simulink model "Flyback Simulink Model"  (R2019b)
settings: Solver=VariableStepAuto  StartTime=0.0  StopTime=5  FixedStep=0.0001  RelTol=1e-3
undefined symbols (not defined in the file): plecs
libraries: simulink x6, plecslib_extras2 x3, simulink_extras x2
settings Model: Creator=jeffl  LastModifiedBy=jeffl
settings SolverCC: ZeroCrossAlgorithm=Adaptive
settings DebuggingCC: IgnoredZcDiagnostic=none

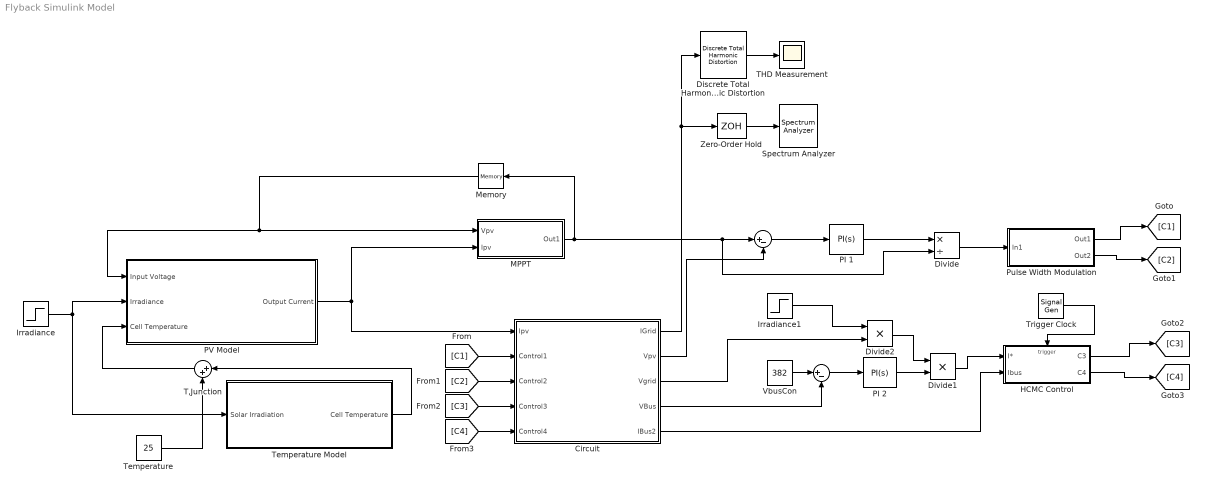
== system Flyback Simulink Model ==
  " " : Sum  Inputs=|+-
  "   " : Sum  Inputs=|+-
  Circuit : Subsystem  LoadFcn=plecs('sl', 200);  InitFcn=plecs('sl', 214);  StartFcn=plecs('sl', 208);  StopFcn=plecs('sl', 209);  mask(PlecsCircuit){PLECSData=<binary blob, 6696 chars, not shown>}
      mask prompts: PLECSData "PLECS Data (Do not delete or modify!)"
      mask init:
      | % PLACE CUSTOM INITIALIZATIONS ABOVE
      | % DO NOT REMOVE
      | plecs('sl', 215);
      | % DO NOT REMOVE
      settings: CopyFcn=plecs('sl', 203);  DeleteFcn=plecs('sl', 205);  UndoDeleteFcn=plecs('sl', 206);  PreSaveFcn=plecs('sl', 211);  PostSaveFcn=plecs('sl', 201);  NameChangeFcn=plecs('sl', 210);  DestroyFcn=plecs('sl', 207);  PreCopyFcn=plecs('sl', 216);  OpenFcn=plecs('sl', 202);  ErrorFcn=plerrorfcn
      mask Help: web(['file:///' fullfile(plecsdoc, 'creatingacircuit.html')])
      mask Display: disp('PLECS\nCircuit')
  Discrete Total Harmonic Distortion : plecslib_extras2/Discrete Analysis/Discrete Total Harmonic Distortion  Ts=1/600  samples=10
      settings: SourceProductName=PLECS Extras
  Divide : Product  Inputs=*/
  Divide1 : Product  Inputs=**
  Divide2 : Product  Inputs=**
  HCMC Control : Subsystem
  Irradiance : Step  Before=1000  After=1000  SampleTime=0
  Irradiance1 : Step  Before=1/220  After=1/245  SampleTime=0
  MPPT : Subsystem
  Memory : Memory  InitialCondition=28
  PI 1 : simulink/Continuous/PID Controller  Controller=PI  Form=Parallel  TimeDomain=Continuous-time  SampleTime=-1  IntegratorMethod=Forward Euler  FilterMethod=Forward Euler  ControllerParametersSource=internal  P=-2  I=-2  D=0  UseFilter=on  N=100  TunerSelectOption=Transfer Function Based (PID Tuner App)  InitialConditionSource=internal  InitialConditionForIntegrator=0  InitialConditionForFilter=0  DifferentiatorICPrevScaledInput=0  ExternalReset=none  TrackingMode=off  Kt=1  LimitOutput=off  UpperSaturationLimit=inf  LowerSaturationLimit=-inf  LinearizeAsGain=on  AntiWindupMode=none  Kb=1  POutMin=[]  POutMax=[]  IOutMin=[]  IOutMax=[]  DOutMin=[]  DOutMax=[]  NOutMin=[]  NOutMax=[]  SumOutMin=[]  SumOutMax=[]  SaturationOutMin=[]  SaturationOutMax=[]  PParamMin=[]  PParamMax=[]  IParamMin=[]  IParamMax=[]  DParamMin=[]  DParamMax=[]  NParamMin=[]  NParamMax=[]  KbParamMin=[]  KbParamMax=[]  KtParamMin=[]  KtParamMax=[]  KbOutMin=[]  KbOutMax=[]  KtOutMin=[]  KtOutMax=[]  IntegratorOutMin=[]  IntegratorOutMax=[]  FilterOutMin=[]  FilterOutMax=[]  SumI1OutMin=[]  SumI1OutMax=[]  SumI2OutMin=[]  SumI2OutMax=[]  SumI3OutMin=[]  SumI3OutMax=[]  SumI4OutMin=[]  SumI4OutMax=[]  SumDOutMin=[]  SumDOutMax=[]  DifferentiatorOutMin=[]  DifferentiatorOutMax=[]  FilterDiffOutCoefMin=[]  FilterDiffOutCoefMax=[]  ReciprocalOutMin=[]  ReciprocalOutMax=[]  SumDenOutMin=[]  SumDenOutMax=[]  SumNumOutMin=[]  SumNumOutMax=[]  DivideOutMin=[]  DivideOutMax=[]  IntegratorContinuousStateAttributes=''  IntegratorStateMustResolveToSignalObject=off  IntegratorRTWStateStorageClass=Auto  FilterContinuousStateAttributes=''  FilterStateMustResolveToSignalObject=off  FilterRTWStateStorageClass=Auto  ParallelPVariant=InternalParameters  IdealPVariant=Disabled  IVariant=InternalParameters  DVariant=Disabled  IntegratorVariant=Continuous  SatVariant=Disabled  AWVariant=Passthrough  PCopyVariant=Disabled  TRVariant=Disabled  FdbkBlocksVariant=Forward  IdealPFdbkVariant=Disabled  SatFdbkVariant=Disabled  DerivativeFilterVariant=Disabled  NVariant=Disabled  NCopyVariant=Disabled_SignalSpec  FilterICVariant=Disabled  IntegratorICVariant=InternalICs  ExternalResetVariant=Disabled  TRSumVariant=Passthrough  SumFdbkVariant=Disabled  SumVariant=Sum_PI
  PI 2 : simulink/Continuous/PID Controller  Controller=PI  Form=Parallel  TimeDomain=Continuous-time  SampleTime=-1  IntegratorMethod=Forward Euler  FilterMethod=Forward Euler  ControllerParametersSource=internal  P=1/10  I=0.5  D=0  UseFilter=on  N=100  TunerSelectOption=Transfer Function Based (PID Tuner App)  InitialConditionSource=internal  InitialConditionForIntegrator=0  InitialConditionForFilter=0  DifferentiatorICPrevScaledInput=0  ExternalReset=none  TrackingMode=off  Kt=1  LimitOutput=off  UpperSaturationLimit=inf  LowerSaturationLimit=-inf  LinearizeAsGain=on  AntiWindupMode=none  Kb=1  POutMin=[]  POutMax=[]  IOutMin=[]  IOutMax=[]  DOutMin=[]  DOutMax=[]  NOutMin=[]  NOutMax=[]  SumOutMin=[]  SumOutMax=[]  SaturationOutMin=[]  SaturationOutMax=[]  PParamMin=[]  PParamMax=[]  IParamMin=[]  IParamMax=[]  DParamMin=[]  DParamMax=[]  NParamMin=[]  NParamMax=[]  KbParamMin=[]  KbParamMax=[]  KtParamMin=[]  KtParamMax=[]  KbOutMin=[]  KbOutMax=[]  KtOutMin=[]  KtOutMax=[]  IntegratorOutMin=[]  IntegratorOutMax=[]  FilterOutMin=[]  FilterOutMax=[]  SumI1OutMin=[]  SumI1OutMax=[]  SumI2OutMin=[]  SumI2OutMax=[]  SumI3OutMin=[]  SumI3OutMax=[]  SumI4OutMin=[]  SumI4OutMax=[]  SumDOutMin=[]  SumDOutMax=[]  DifferentiatorOutMin=[]  DifferentiatorOutMax=[]  FilterDiffOutCoefMin=[]  FilterDiffOutCoefMax=[]  ReciprocalOutMin=[]  ReciprocalOutMax=[]  SumDenOutMin=[]  SumDenOutMax=[]  SumNumOutMin=[]  SumNumOutMax=[]  DivideOutMin=[]  DivideOutMax=[]  IntegratorContinuousStateAttributes=''  IntegratorStateMustResolveToSignalObject=off  IntegratorRTWStateStorageClass=Auto  FilterContinuousStateAttributes=''  FilterStateMustResolveToSignalObject=off  FilterRTWStateStorageClass=Auto  ParallelPVariant=InternalParameters  IdealPVariant=Disabled  IVariant=InternalParameters  DVariant=Disabled  IntegratorVariant=Continuous  SatVariant=Disabled  AWVariant=Passthrough  PCopyVariant=Disabled  TRVariant=Disabled  FdbkBlocksVariant=Forward  IdealPFdbkVariant=Disabled  SatFdbkVariant=Disabled  DerivativeFilterVariant=Disabled  NVariant=Disabled  NCopyVariant=Disabled_SignalSpec  FilterICVariant=Disabled  IntegratorICVariant=InternalICs  ExternalResetVariant=Disabled  TRSumVariant=Passthrough  SumFdbkVariant=Disabled  SumVariant=Sum_PI
  PV Model : Subsystem
  Pulse Width Modulation : Subsystem
  "Spectrum Analyzer " : SpectrumAnalyzer
  T,Junction : Sum  Inputs=|++
  THD Measurement : Scope
  Temperature : Constant  Value=25
  Temperature Model : Subsystem
  Trigger Clock : SignalGenerator  WaveForm=square  Frequency=400e3  Units=rad/sec
  VbusCon : Constant  Value=382
  Zero-Order Hold : ZeroOrderHold  SampleTime=1/1500
  wires:
  MPPT/1(Out1) -> Memory/1, Divide/2, " "/1
  Memory/1 -> PV Model/1(Input Voltage), MPPT/1(Vpv)
  PV Model/1(Output Current) -> MPPT/2(Ipv), Circuit/1(Ipv)
  T,Junction/1 -> PV Model/3(Cell Temperature)
  Temperature/1 -> T,Junction/2
  Temperature Model/1(Cell Temperature) -> T,Junction/1
  Irradiance/1 -> PV Model/2(Irradiance), Temperature Model/1(Solar Irradiation)
  " "/1 -> PI 1/1
  PI 1/1 -> Divide/1
  Divide/1 -> Pulse Width Modulation/1(In1)
  Circuit/2(Vpv) -> " "/2
  Circuit/4(VBus) -> "   "/2
  VbusCon/1 -> "   "/1
  "   "/1 -> PI 2/1
  PI 2/1 -> Divide1/2
  Divide1/1 -> HCMC Control/1(I*)
  Circuit/5(IBus2) -> HCMC Control/2(Ibus)
  Trigger Clock/1 -> HCMC Control/Trigger
  Circuit/1(IGrid) -> Discrete Total Harmonic Distortion/1, Zero-Order Hold/1
  Discrete Total Harmonic Distortion/1 -> THD Measurement/1
  Zero-Order Hold/1 -> "Spectrum Analyzer "/1
  Pulse Width Modulation/1(Out1) -> [C1]
  Pulse Width Modulation/2(Out2) -> [C2]
  [C1] -> Circuit/2(Control1)
  [C2] -> Circuit/3(Control2)
  HCMC Control/2(C4) -> [C4]
  HCMC Control/1(C3) -> [C3]
  [C4] -> Circuit/5(Control4)
  [C3] -> Circuit/4(Control3)
  Circuit/3(Vgrid) -> Divide2/2
  Irradiance1/1 -> Divide2/1
  Divide2/1 -> Divide1/1

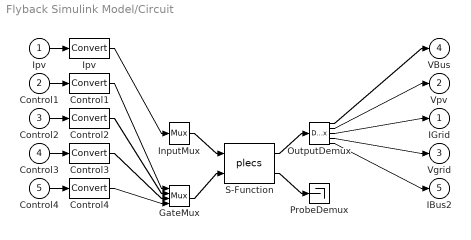
== system Flyback Simulink Model/Circuit ==
  Ipv : Inport  PortDimensions=1
  Control1 : Inport  Port=2  PortDimensions=1
  Control2 : Inport  Port=3  PortDimensions=1
  Control3 : Inport  Port=4  PortDimensions=1
  Control4 : Inport  Port=5  PortDimensions=1
  " Control1 " : DataTypeConversion  SaturateOnIntegerOverflow=on  RndMeth=Zero
  " Control2 " : DataTypeConversion  SaturateOnIntegerOverflow=on  RndMeth=Zero
  " Control3 " : DataTypeConversion  SaturateOnIntegerOverflow=on  RndMeth=Zero
  " Control4 " : DataTypeConversion  SaturateOnIntegerOverflow=on  RndMeth=Zero
  " GateMux " : Mux  Inputs=[ 1 1 1 1 ]
  " InputMux " : Mux  Inputs=[ 1 ]
  " Ipv " : DataTypeConversion  SaturateOnIntegerOverflow=on  RndMeth=Zero
  " OutputDemux " : Demux  Outputs=[ 1 1 1 1 1 ]
  " ProbeDemux " : Terminator
  " S-Function " : S-Function  FunctionName=plecs  SFunctionDeploymentMode=off  EnableBusSupport=off
  IGrid : Outport  PortDimensions=1
  Vpv : Outport  Port=2  PortDimensions=1
  Vgrid : Outport  Port=3  PortDimensions=1
  VBus : Outport  Port=4  PortDimensions=1
  IBus2 : Outport  Port=5  PortDimensions=1
  wires:
  " InputMux "/1 -> " S-Function "/1
  " GateMux "/1 -> " S-Function "/2
  " S-Function "/1 -> " OutputDemux "/1
  " S-Function "/2 -> " ProbeDemux "/1
  Ipv/1 -> " Ipv "/1
  " Ipv "/1 -> " InputMux "/1
  Control1/1 -> " Control1 "/1
  " Control1 "/1 -> " GateMux "/1
  Control2/1 -> " Control2 "/1
  " Control2 "/1 -> " GateMux "/2
  Control3/1 -> " Control3 "/1
  " Control3 "/1 -> " GateMux "/3
  Control4/1 -> " Control4 "/1
  " Control4 "/1 -> " GateMux "/4
  " OutputDemux "/1 -> VBus/1
  " OutputDemux "/2 -> Vpv/1
  " OutputDemux "/3 -> IGrid/1
  " OutputDemux "/4 -> Vgrid/1
  " OutputDemux "/5 -> IBus2/1

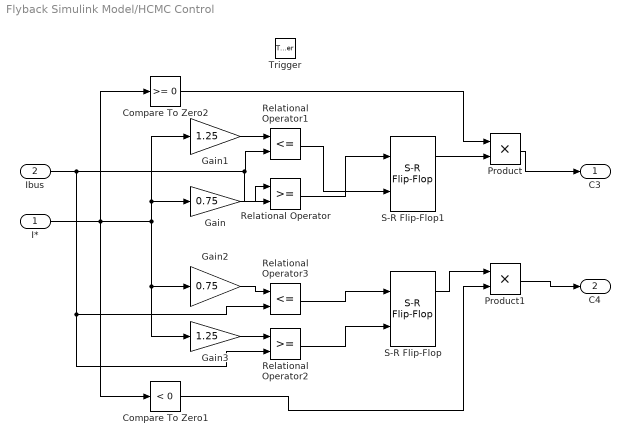
== system Flyback Simulink Model/HCMC Control ==
  I* : Inport
  Ibus : Inport  Port=2
  Trigger : TriggerPort  VariantControl=Variant  PortDimensions=1
  Compare To Zero1 : simulink/Logic and Bit Operations/Compare To Zero  relop=<  OutDataTypeStr=boolean  ZeroCross=off
  Compare To Zero2 : simulink/Logic and Bit Operations/Compare To Zero  relop=>=  OutDataTypeStr=boolean  ZeroCross=off
  Gain : Gain  Gain=0.75
  Gain1 : Gain  Gain=1.25
  Gain2 : Gain  Gain=0.75
  Gain3 : Gain  Gain=1.25
  Product : Product
  Product1 : Product
  Relational Operator : RelationalOperator  OutDataTypeStr=boolean  ZeroCross=off  RndMeth=Simplest
  Relational Operator1 : RelationalOperator  Operator=<=  OutDataTypeStr=boolean  ZeroCross=off  RndMeth=Simplest
  Relational Operator2 : RelationalOperator  OutDataTypeStr=boolean  ZeroCross=off  RndMeth=Simplest
  Relational Operator3 : RelationalOperator  Operator=<=  OutDataTypeStr=boolean  ZeroCross=off  RndMeth=Simplest
  S-R Flip-Flop : simulink_extras/Flip Flops/S-R Flip-Flop  initial_condition=0
  S-R Flip-Flop1 : simulink_extras/Flip Flops/S-R Flip-Flop  initial_condition=0
  C3 : Outport
  C4 : Outport  Port=2
  wires:
  I*/1 -> Gain3/1, Gain2/1, Gain1/1, Gain/1, Compare To Zero1/1, Compare To Zero2/1
  Gain1/1 -> Relational Operator1/1
  Compare To Zero2/1 -> Product/1
  Compare To Zero1/1 -> Product1/2
  S-R Flip-Flop/1 -> Product1/1
  S-R Flip-Flop1/1 -> Product/2
  Product/1 -> C3/1
  Product1/1 -> C4/1
  Ibus/1 -> Relational Operator/2, Relational Operator1/2, Relational Operator3/2, Relational Operator2/2
  Gain/1 -> Relational Operator/1
  Gain3/1 -> Relational Operator2/1
  Gain2/1 -> Relational Operator3/1
  Relational Operator/1 -> S-R Flip-Flop1/1
  Relational Operator1/1 -> S-R Flip-Flop1/2
  Relational Operator3/1 -> S-R Flip-Flop/1
  Relational Operator2/1 -> S-R Flip-Flop/2

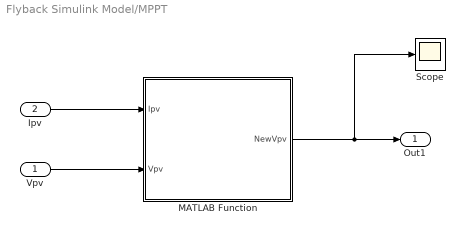
== system Flyback Simulink Model/MPPT ==
  Vpv : Inport
  Ipv : Inport  Port=2
  MATLAB Function : MATLAB Function  TreatAsAtomicUnit=on
  Scope : Scope
  Out1 : Outport  VectorParamsAs1DForOutWhenUnconnected=off
  wires:
  Ipv/1 -> MATLAB Function/1(Ipv)
  Vpv/1 -> MATLAB Function/2(Vpv)
  MATLAB Function/1(NewVpv) -> Scope/1, Out1/1

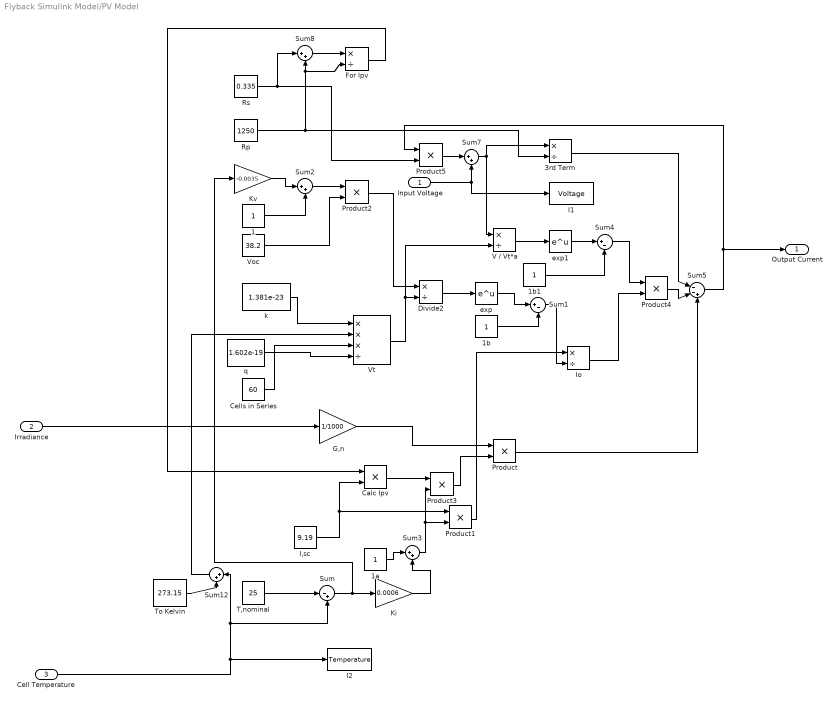
== system Flyback Simulink Model/PV Model ==
  Input Voltage : Inport
  Irradiance : Inport  Port=2
  Cell Temperature : Inport  Port=3
  1 : Constant
  1a : Constant
  1b : Constant
  1b1 : Constant
  3rd Term : Product  Inputs=*/
  Calc Ipv : Product
  Cells in Series : Constant  Value=60
  Divide2 : Product  Inputs=*/
  For Ipv : Product  Inputs=*/
  G,n : Gain  Gain=1/1000
  I,sc : Constant  Value=9.19
  I1 : ToWorkspace  VariableName=Voltage  SampleTime=-1
  I2 : ToWorkspace  VariableName=Temperature  SampleTime=-1
  Io : Product  Inputs=*/
  Ki : Gain  Gain=0.0006
  Kv : Gain  Gain=-0.0035
  Product{,1..5} (6 alike) : Product
  Rp : Constant  Value=1250
  Rs : Constant  Value=0.335
  Sum : Sum  Inputs=|-+
  Sum1 : Sum  Inputs=|+-
  Sum{2..3,7..8,12} (5 alike) : Sum  Inputs=|++
  Sum4 : Sum  Inputs=|+-
  Sum5 : Sum  Inputs=|--+
  T,nominal : Constant  Value=25
  To Kelvin : Constant  Value=273.15
  V / Vt*a : Product  Inputs=*/
  Voc : Constant  Value=38.2
  Vt : Product  Inputs=***/
  exp : Math  SaturateOnIntegerOverflow=on
  exp1 : Math  SaturateOnIntegerOverflow=on
  k : Constant  Value=1.381e-23
  q : Constant  Value=1.602e-19
  Output Current : Outport  VectorParamsAs1DForOutWhenUnconnected=off
  wires:
  1b1/1 -> Sum4/2
  I,sc/1 -> Product1/1, Calc Ipv/2
  Io/1 -> Product4/2
  Ki/1 -> Sum3/2
  exp/1 -> Sum1/1
  For Ipv/1 -> Calc Ipv/1
  3rd Term/1 -> Sum5/1
  Input Voltage/1 -> Sum7/2, I1/1
  To Kelvin/1 -> Sum12/2
  Sum7/1 -> V / Vt*a/1, 3rd Term/1
  Product2/1 -> Divide2/1
  Product/1 -> Sum5/3
  1/1 -> Sum2/2
  Rp/1 -> For Ipv/2, Sum8/2, 3rd Term/2
  Calc Ipv/1 -> Product3/1
  Product4/1 -> Sum5/2
  Sum1/1 -> Io/2
  Sum8/1 -> For Ipv/1
  1b/1 -> Sum1/2
  Sum12/1 -> Vt/2
  Divide2/1 -> exp/1
  V / Vt*a/1 -> exp1/1
  Voc/1 -> Product2/2
  Sum2/1 -> Product2/1
  Kv/1 -> Sum2/1
  1a/1 -> Sum3/1
  Cell Temperature/1 -> I2/1, Sum/2, Sum12/1
  Product3/1 -> Product/2
  G,n/1 -> Product/1
  k/1 -> Vt/1
  T,nominal/1 -> Sum/1
  Irradiance/1 -> G,n/1
  Rs/1 -> Sum8/1, Product5/2
  Sum3/1 -> Product1/2, Product3/2
  Sum/1 -> Kv/1, Ki/1
  Product5/1 -> Sum7/1
  Sum5/1 -> Output Current/1, Product5/1
  Vt/1 -> V / Vt*a/2, Divide2/2
  q/1 -> Vt/4
  Cells in Series/1 -> Vt/3
  Product1/1 -> Io/1
  exp1/1 -> Sum4/1
  Sum4/1 -> Product4/1

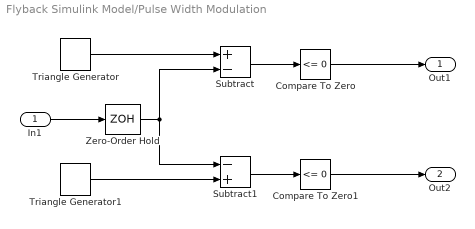
== system Flyback Simulink Model/Pulse Width Modulation ==
  In1 : Inport
  Compare To Zero : simulink/Logic and Bit Operations/Compare To Zero  relop=<=  OutDataTypeStr=boolean
  Compare To Zero1 : simulink/Logic and Bit Operations/Compare To Zero  relop=<=  OutDataTypeStr=boolean
  Subtract : Sum  Inputs=+-
  Subtract1 : Sum  Inputs=-+
  Triangle Generator : plecslib_extras2/Modulators/Triangle Generator  fc=10e3  offset=0  range=[0 1]
      settings: SourceProductName=PLECS Extras
  Triangle Generator1 : plecslib_extras2/Modulators/Triangle Generator  fc=10e3  offset=.5  range=[0 1]
      settings: SourceProductName=PLECS Extras
  Zero-Order Hold : ZeroOrderHold  SampleTime=-1
  Out1 : Outport
  Out2 : Outport  Port=2
  wires:
  Triangle Generator/1 -> Subtract/1
  Zero-Order Hold/1 -> Subtract/2, Subtract1/1
  Triangle Generator1/1 -> Subtract1/2
  Subtract/1 -> Compare To Zero/1
  Subtract1/1 -> Compare To Zero1/1
  Compare To Zero/1 -> Out1/1
  Compare To Zero1/1 -> Out2/1
  In1/1 -> Zero-Order Hold/1

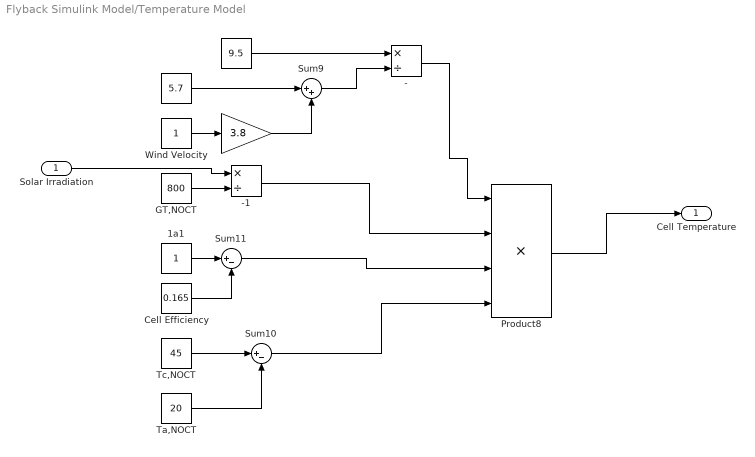
== system Flyback Simulink Model/Temperature Model ==
  Solar Irradiation : Inport
  " " : Constant  Value=5.7
  "  " : Gain  Gain=3.8
  "    " : Constant  Value=9.5
  - : Product  Inputs=*/
  -1 : Product  Inputs=*/
  1a1 : Constant
  Cell Efficiency : Constant  Value=0.165
  GT,NOCT : Constant  Value=800
  Product8 : Product  Inputs=4
  Sum10 : Sum  Inputs=|+-
  Sum11 : Sum  Inputs=|+-
  Sum9 : Sum  Inputs=|++
  Ta,NOCT : Constant  Value=20
  Tc,NOCT : Constant  Value=45
  Wind Velocity : Constant
  Cell Temperature : Outport  VectorParamsAs1DForOutWhenUnconnected=off
  wires:
  GT,NOCT/1 -> -1/2
  Sum10/1 -> Product8/4
  "    "/1 -> -/1
  Ta,NOCT/1 -> Sum10/2
  Sum9/1 -> -/2
  Wind Velocity/1 -> "  "/1
  " "/1 -> Sum9/1
  Tc,NOCT/1 -> Sum10/1
  -/1 -> Product8/1
  "  "/1 -> Sum9/2
  Product8/1 -> Cell Temperature/1
  -1/1 -> Product8/2
  1a1/1 -> Sum11/1
  Cell Efficiency/1 -> Sum11/2
  Sum11/1 -> Product8/3
  Solar Irradiation/1 -> -1/1

== matlab function Flyback Simulink Model/MPPT/MATLAB Function ==
  settings: updateMethod=DISCRETE
  data: Ipv input; Vpv input; NewVpv output
function NewVpv = PerturbObserve(Ipv,Vpv)

persistent Pprev Vprev Dprev M,

M = 0.000555;

if isempty(Dprev)
    Dprev = 0.1;
    Vprev = 32.1;
    Pprev = 130;
end

Ppv = Ipv * Vpv;
Slope = (Ppv - Pprev)/(Vpv-Vprev);
if abs(Slope) > 50
    if Slope > 0
        Slope = 5;
    else 
        Slope = -5;
    end 
end 

if abs(Ppv - Pprev) >= 1e-8
    if (Ppv-Pprev) > 0
        if (Vpv-Vprev) > 0
            D = M * Slope;
            NewVpv = (1+D) * Vpv;
         
        else
            D = M * Slope;
            NewVpv = (1+D) * Vpv;

        end
    else
        if (Vpv-Vprev) > 0
            D = M * Slope;
            NewVpv = (1+D) * Vpv;
            
        else
            D = M * Slope;
            NewVpv = (1+D) * Vpv;

        end        
    end
    
    
else

    Vprev = 32;
    D = 0;
    NewVpv = (1+D) * Vpv;
end    

Dprev = D;

if NewVpv > 35
    NewVpv = 30;
elseif Vprev ~=32
    Vprev = Vpv;
end 

    
Pprev = Ppv;
